simulink model "test_model"  (R2022b)
settings: Solver=VariableStepAuto  StartTime=0.0  StopTime=7  RelTol=1e-3
values from neighbouring files (symbols this model uses):
  A = 1.08    [test_script.m]
  b = 0.1    [test_script.m]
  c = 0.008    [test_script.m]
  Cd = 1.02    [test_script.m]
  g = 9.81    [test_script.m]
  gr = 47/13    (= 3.61538461538)    [test_script.m]
  h_cg = .259    (= 0.259)    [test_script.m]
  h_d = h_cg    (= 0.259)    [test_script.m]
  J = 0.27    [test_script.m]
  m = 297    [test_script.m]
  r = 0.5588    [test_script.m]
  rho = 1.162    [test_script.m]
  wb = 1.53    [test_script.m]
  wb_f = 0.813    [test_script.m]
libraries: dspswit3 x2, slpidlib x1
settings Model: Creator=sahil  LastModifiedBy=PC
settings ModelReferenceCC: EnableRefExpFcnMdlSchedulingChecks=on

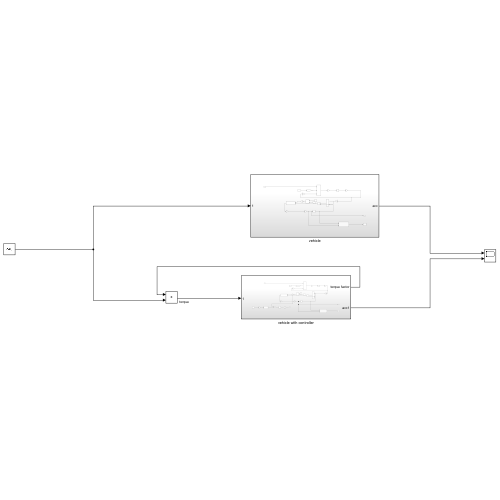
[thumbnail: Simulink's stored preview of the top-level diagram]
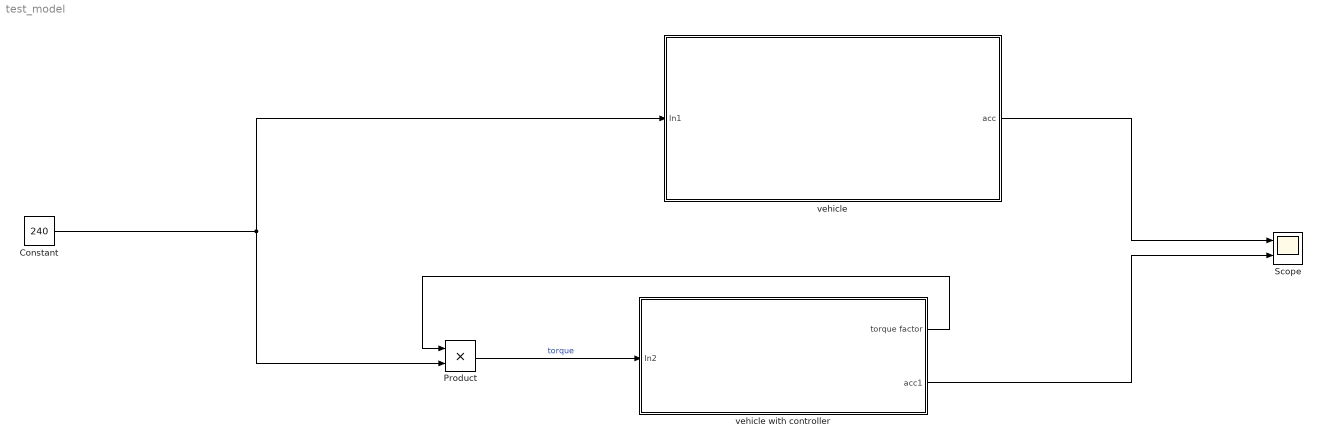
== system test_model ==
  Constant : Constant  Value=240
  Product : Product
  Scope : Scope  NumInputPorts=2
  vehicle : Subsystem
  vehicle with controller : Subsystem
  wires:
  Constant/1 -> vehicle/1(In1), Product/2
  vehicle/1(acc) -> Scope/1
  vehicle with controller/2(acc1) -> Scope/2
  Product/1 -> vehicle with controller/1(In2)  "torque"
  vehicle with controller/1(torque factor) -> Product/1

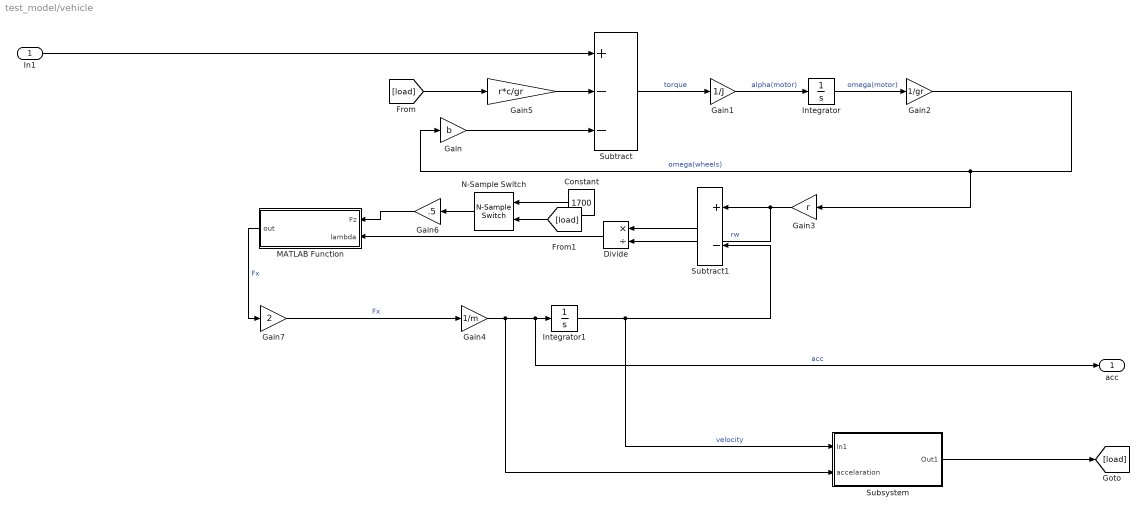
== system test_model/vehicle ==
  In1 : Inport
  Constant : Constant  Value=1700
  Divide : Product  Inputs=*/
  Gain : Gain  Gain=b
  Gain1 : Gain  Gain=1/J
  Gain2 : Gain  Gain=1/gr
  Gain3 : Gain  Gain=r
  Gain4 : Gain  Gain=1/m
  Gain5 : Gain  Gain=r*c/gr
  Gain6 : Gain  Gain=.5
  Gain7 : Gain  Gain=2
  Integrator : Integrator  InitialCondition=86.13
  Integrator1 : Integrator  InitialCondition=1
  MATLAB Function : MATLAB Function  TreatAsAtomicUnit=on
  N-Sample Switch : dspswit3/N-Sample Switch  N=1  reset=off  TriggerType=Rising edge  Ts=0.1
  Subsystem : Subsystem
  Subtract : Sum  Inputs=+--
  Subtract1 : Sum  Inputs=+-
  acc : Outport
  wires:
  Gain3/1 -> Divide/2, Subtract1/1  "rw"
  Gain/1 -> Subtract/3
  Subtract/1 -> Gain1/1  "torque"
  Gain5/1 -> Subtract/2
  Gain2/1 -> Gain3/1, Gain/1  "omega(wheels)"
  Integrator/1 -> Gain2/1  "omega(motor)"
  [load] -> Gain5/1
  Gain1/1 -> Integrator/1  "alpha(motor)"
  Integrator1/1 -> Subsystem/1(In1), Subtract1/2  "velocity"
  Divide/1 -> MATLAB Function/2(lambda)
  Subtract1/1 -> Divide/1
  Gain4/1 -> Subsystem/2(accelaration), acc/1, Integrator1/1  "acc"
  Gain7/1 -> Gain4/1  "Fx"
  Subsystem/1(Out1) -> [load]
  In1/1 -> Subtract/1
  MATLAB Function/1(out) -> Gain7/1  "Fx"
  Constant/1 -> N-Sample Switch/1
  [load] -> N-Sample Switch/2
  N-Sample Switch/1 -> Gain6/1
  Gain6/1 -> MATLAB Function/1(Fz)

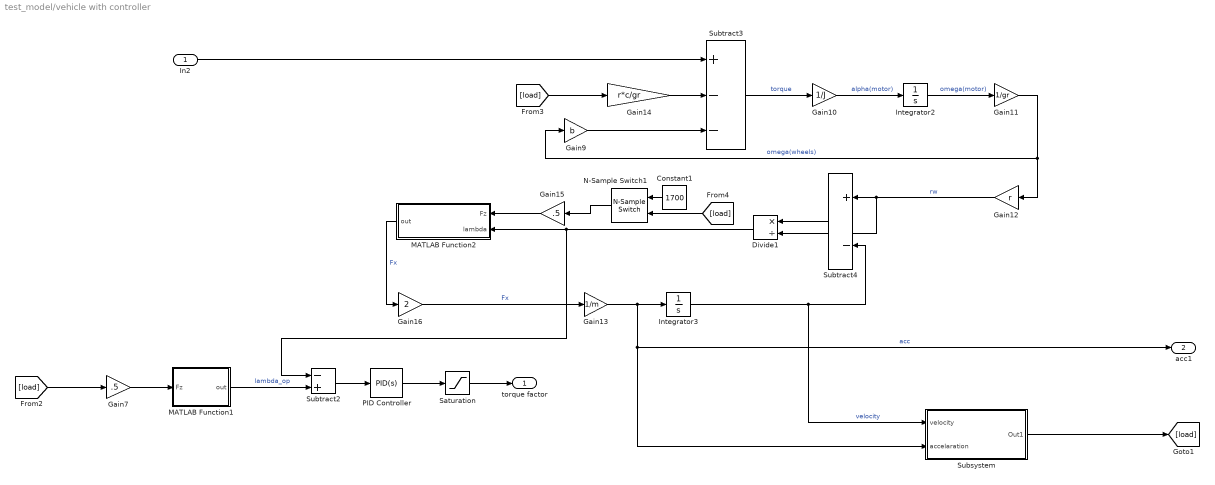
== system test_model/vehicle with controller ==
  In2 : Inport
  Constant1 : Constant  Value=1700
  Divide1 : Product  Inputs=*/
  Gain10 : Gain  Gain=1/J
  Gain11 : Gain  Gain=1/gr
  Gain12 : Gain  Gain=r
  Gain13 : Gain  Gain=1/m
  Gain14 : Gain  Gain=r*c/gr
  Gain15 : Gain  Gain=.5
  Gain16 : Gain  Gain=2
  Gain7 : Gain  Gain=.5
  Gain9 : Gain  Gain=b
  Integrator2 : Integrator  InitialCondition=86.13
  Integrator3 : Integrator  InitialCondition=1
  MATLAB Function1 : MATLAB Function  TreatAsAtomicUnit=on
  MATLAB Function2 : MATLAB Function  TreatAsAtomicUnit=on
  N-Sample Switch1 : dspswit3/N-Sample Switch  N=1  reset=off  TriggerType=Rising edge  Ts=0.1
  PID Controller : slpidlib/PID Controller  Controller=PID  Form=Parallel  TimeDomain=Continuous-time  UseExternalTs=off  SampleTime=-1  IntegratorMethod=Forward Euler  FilterMethod=Forward Euler  ControllerParametersSource=internal  P=0  I=0  UseKiTs=off  D=162.3542  N=30  UseFilter=on  TunerSelectOption=Frequency Response Based  InitialConditionSource=internal  InitialConditionForIntegrator=0  InitialConditionForFilter=0  DifferentiatorICPrevScaledInput=0  ExternalReset=none  TrackingMode=off  Kt=1  LimitOutput=off  SatLimitsSource=internal  UpperSaturationLimit=inf  LowerSaturationLimit=-inf  LinearizeAsGain=on  AntiWindupMode=none  Kb=1  LimitIntegrator=off  UpperIntegratorSaturationLimit=inf  LowerIntegratorSaturationLimit=-inf  POutMin=[]  POutMax=[]  IOutMin=[]  IOutMax=[]  DOutMin=[]  DOutMax=[]  NOutMin=[]  NOutMax=[]  SumOutMin=[]  SumOutMax=[]  SaturationOutMin=[]  SaturationOutMax=[]  PParamMin=[]  PParamMax=[]  IParamMin=[]  IParamMax=[]  DParamMin=[]  DParamMax=[]  NParamMin=[]  NParamMax=[]  KbParamMin=[]  KbParamMax=[]  KtParamMin=[]  KtParamMax=[]  KbOutMin=[]  KbOutMax=[]  KtOutMin=[]  KtOutMax=[]  IntegratorOutMin=[]  IntegratorOutMax=[]  FilterOutMin=[]  FilterOutMax=[]  SumI1OutMin=[]  SumI1OutMax=[]  SumI2OutMin=[]  SumI2OutMax=[]  SumI3OutMin=[]  SumI3OutMax=[]  SumI4OutMin=[]  SumI4OutMax=[]  SumDOutMin=[]  SumDOutMax=[]  DifferentiatorOutMin=[]  DifferentiatorOutMax=[]  FilterDiffOutCoefMin=[]  FilterDiffOutCoefMax=[]  ReciprocalOutMin=[]  ReciprocalOutMax=[]  SumDenOutMin=[]  SumDenOutMax=[]  SumNumOutMin=[]  SumNumOutMax=[]  DivideOutMin=[]  DivideOutMax=[]  UdiffTsProdOutMin=[]  UdiffTsProdOutMax=[]  NTsProdOutMin=[]  NTsProdOutMax=[]  UintegralTsProdOutMin=[]  UintegralTsProdOutMax=[]  UngainTsProdOutMin=[]  UngainTsProdOutMax=[]  ClampingZeroOutDataTypeStr=Inherit: Inherit via back propagation  ClampingZeroOutMin=[]  ClampingZeroOutMax=[]  FilterDenConstantOutDataTypeStr=Inherit: Inherit via back propagation  FilterDenConstantOutMin=[]  FilterDenConstantOutMax=[]  PCopyOutDataTypeStr=Inherit: Inherit via back propagation  PCopyOutMin=[]  PCopyOutMax=[]  NCopyOutDataTypeStr=Inherit: Inherit via back propagation  NCopyOutMin=[]  NCopyOutMax=[]  IntegratorContinuousStateAttributes=''  IntegratorStateMustResolveToSignalObject=off  IntegratorRTWStateStorageClass=Auto  FilterContinuousStateAttributes=''  FilterStateMustResolveToSignalObject=off  FilterRTWStateStorageClass=Auto  ParallelPVariant=InternalParameters  IdealPVariant=Disabled  IVariant=InternalParameters  DVariant=InternalParameters  IntegratorVariant=Continuous  SatVariant=Disabled  AWVariant=Passthrough  PCopyVariant=Disabled  TRVariant=Disabled  FdbkBlocksVariant=Forward  IdealPFdbkVariant=Disabled  SatFdbkVariant=Disabled  DerivativeFilterVariant=ContFilter  NVariant=InternalParameters  NCopyVariant=Disabled  FilterICVariant=InternalICsFilter  IntegratorICVariant=InternalICs  ExternalResetVariant=Disabled  TRSumVariant=Passthrough  SumFdbkVariant=Disabled  SumVariant=Sum_PID  TsampFilterVariant=InternalTs  TsampNgainVariant=Passthrough  TsampIntegralVariant=Passthrough  ExternalSaturationOutDataTypeStr=Inherit: Same as second input
  Saturation : Saturate  UpperLimit=1  LowerLimit=0
  Subsystem : Subsystem
  Subtract2 : Sum  Inputs=-+
  Subtract3 : Sum  Inputs=+--
  Subtract4 : Sum  Inputs=+-
  torque factor : Outport
  acc1 : Outport  Port=2
  wires:
  [load] -> Gain7/1
  MATLAB Function1/1(out) -> Subtract2/2  "lambda_op"
  Saturation/1 -> torque factor/1
  Gain7/1 -> MATLAB Function1/1(Fz)
  N-Sample Switch1/1 -> Gain15/1
  MATLAB Function2/1(out) -> Gain16/1  "Fx"
  [load] -> Gain14/1
  Integrator3/1 -> Subsystem/1(velocity), Subtract4/2  "velocity"
  Gain13/1 -> acc1/1, Subsystem/2(accelaration), Integrator3/1  "acc"
  Subtract4/1 -> Divide1/1
  Divide1/1 -> Subtract2/1, MATLAB Function2/2(lambda)
  Integrator2/1 -> Gain11/1  "omega(motor)"
  Subsystem/1(Out1) -> [load]
  Subtract3/1 -> Gain10/1  "torque"
  In2/1 -> Subtract3/1
  Gain9/1 -> Subtract3/3
  Gain10/1 -> Integrator2/1  "alpha(motor)"
  Gain16/1 -> Gain13/1  "Fx"
  Gain11/1 -> Gain12/1, Gain9/1  "omega(wheels)"
  Gain14/1 -> Subtract3/2
  Gain12/1 -> Divide1/2, Subtract4/1  "rw"
  Gain15/1 -> MATLAB Function2/1(Fz)
  Constant1/1 -> N-Sample Switch1/1
  [load] -> N-Sample Switch1/2
  PID Controller/1 -> Saturation/1
  Subtract2/1 -> PID Controller/1

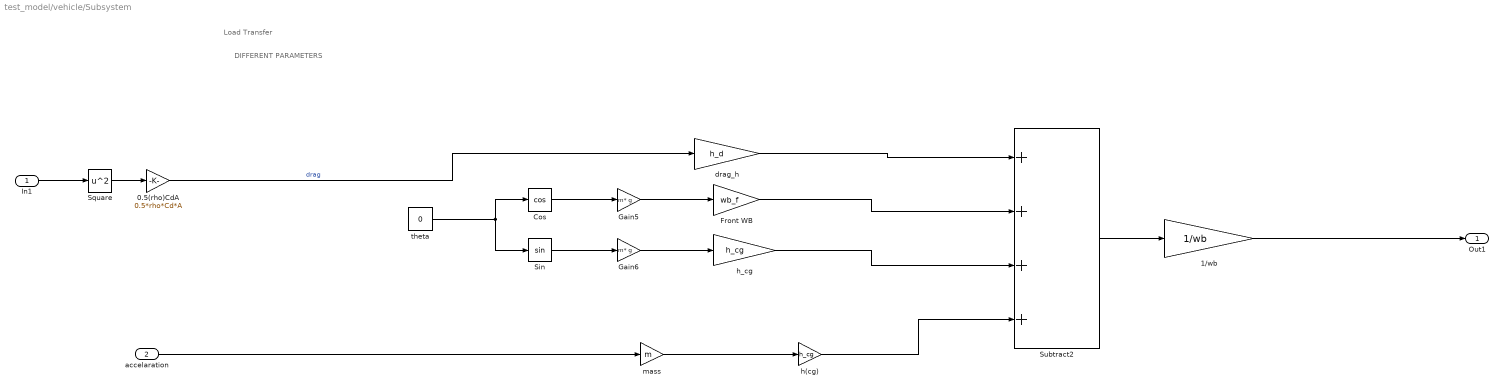
== system test_model/vehicle/Subsystem ==
  note: Load Transfer
  note: DIFFERENT PARAMETERS
  In1 : Inport
  accelaration : Inport  Port=2
  0.5(rho)CdA : Gain  Gain=0.5*rho*Cd*A
  1/wb : Gain  Gain=1/wb
  Cos : Trigonometry  Operator=cos
  Front WB : Gain  Gain=wb_f
  Gain5 : Gain  Gain=m* g
  Gain6 : Gain  Gain=m* g
  Sin : Trigonometry
  Square : Math  Operator=square
  Subtract2 : Sum  Inputs=++++
  drag_h : Gain  Gain=h_d
  h(cg) : Gain  Gain=h_cg
  h_cg : Gain  Gain=h_cg
  mass : Gain  Gain=m
  theta : Constant  Value=0
  Out1 : Outport
  wires:
  Cos/1 -> Gain5/1
  Gain6/1 -> h_cg/1
  theta/1 -> Sin/1, Cos/1
  0.5(rho)CdA/1 -> drag_h/1  "drag"
  Subtract2/1 -> 1/wb/1
  accelaration/1 -> mass/1
  drag_h/1 -> Subtract2/1
  h_cg/1 -> Subtract2/3
  Sin/1 -> Gain6/1
  Gain5/1 -> Front WB/1
  h(cg)/1 -> Subtract2/4
  Front WB/1 -> Subtract2/2
  Square/1 -> 0.5(rho)CdA/1
  mass/1 -> h(cg)/1
  1/wb/1 -> Out1/1
  In1/1 -> Square/1

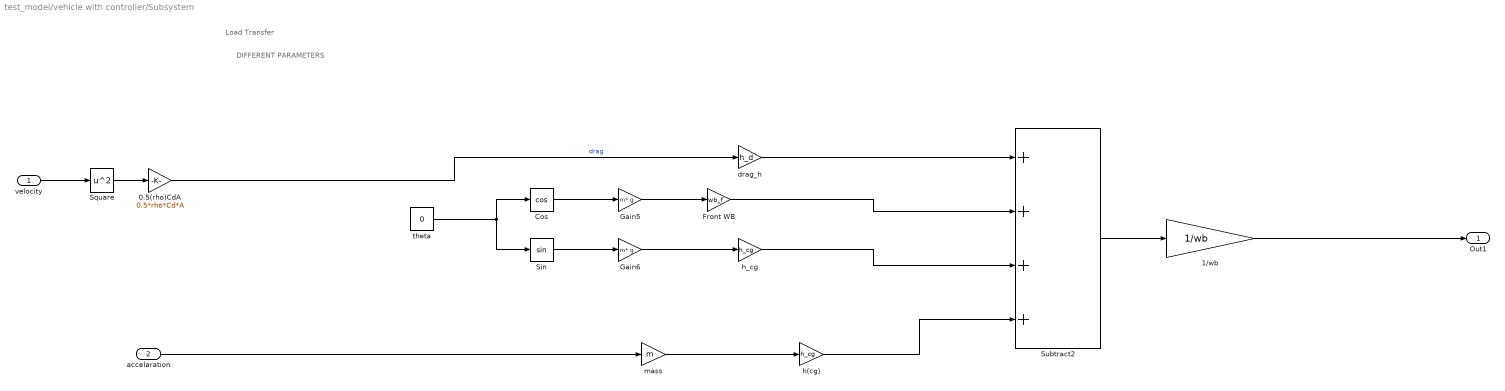
== system test_model/vehicle with controller/Subsystem ==
  note: Load Transfer
  note: DIFFERENT PARAMETERS
  velocity : Inport
  accelaration : Inport  Port=2
  0.5(rho)CdA : Gain  Gain=0.5*rho*Cd*A
  1/wb : Gain  Gain=1/wb
  Cos : Trigonometry  Operator=cos
  Front WB : Gain  Gain=wb_f
  Gain5 : Gain  Gain=m* g
  Gain6 : Gain  Gain=m* g
  Sin : Trigonometry
  Square : Math  Operator=square
  Subtract2 : Sum  Inputs=++++
  drag_h : Gain  Gain=h_d
  h(cg) : Gain  Gain=h_cg
  h_cg : Gain  Gain=h_cg
  mass : Gain  Gain=m
  theta : Constant  Value=0
  Out1 : Outport
  wires:
  Cos/1 -> Gain5/1
  Gain6/1 -> h_cg/1
  theta/1 -> Sin/1, Cos/1
  0.5(rho)CdA/1 -> drag_h/1  "drag"
  Subtract2/1 -> 1/wb/1
  accelaration/1 -> mass/1
  drag_h/1 -> Subtract2/1
  h_cg/1 -> Subtract2/3
  Sin/1 -> Gain6/1
  Gain5/1 -> Front WB/1
  h(cg)/1 -> Subtract2/4
  Front WB/1 -> Subtract2/2
  Square/1 -> 0.5(rho)CdA/1
  mass/1 -> h(cg)/1
  1/wb/1 -> Out1/1
  velocity/1 -> Square/1

== matlab function test_model/vehicle with controller/MATLAB Function1 ==
  data: Fz input; out output
function out=packeja(Fz)
    
    a1=-2.13*(10^-5);
    a2=1.144;
    a3=4.96*(10^-5);
    a4=.226;
    a5=6.9*(10^-5);
    a6=-6*(10^-9);
    a7=5.6*(10*(-5));
    a8=.486;
    
    lambda=0:.005:1;
    Cx=1.65;
    Dx=a1*Fz*Fz+a2*Fz;
    func1=(a3*Fz*Fz+a4*Fz)*exp(-a5*Fz);
    Bx=func1/(Cx*Dx);
    Ex=a6*Fz*Fz+a7*Fz+a8;
    G=Bx*lambda;
    func2=G*(1-Ex)+Ex*atan(G);
    Fx=Dx*sin(Cx*atan(func2));
    plot(lambda,Fx)
    [~,I]=max(Fx);
    slip=lambda(I);
    out=slip;

end

== matlab function test_model/vehicle with controller/MATLAB Function2 ==
  data: Fz input; out output; lambda input
function out=force(Fz,lambda)
    
    
    a1=-2.13*(10^-5);
    a2=1.144;
    a3=4.96*(10^-5);
    a4=.226;
    a5=6.9*(10^-5);
    a6=-6*(10^-9);
    a7=5.6*(10*(-5));
    a8=.486;
    
    
    Cx=1.65;
    Dx=a1*Fz*Fz+a2*Fz;
    func1=(a3*Fz*Fz+a4*Fz)*exp(-a5*Fz);
    Bx=func1/(Cx*Dx);
    Ex=a6*Fz*Fz+a7*Fz+a8;
    G=Bx*lambda;
    func2=G*(1-Ex)+Ex*atan(G);
    Fx=Dx*sin(Cx*atan(func2));
    out = Fx;
end

== matlab function test_model/vehicle/MATLAB Function ==
  data: Fz input; out output; lambda input
function out=force(Fz,lambda)
    
    
    a1=-2.13*(10^-5);
    a2=1.144;
    a3=4.96*(10^-5);
    a4=.226;
    a5=6.9*(10^-5);
    a6=-6*(10^-9);
    a7=5.6*(10*(-5));
    a8=.486;
    
    
    Cx=1.65;
    Dx=a1*Fz*Fz+a2*Fz;
    func1=(a3*Fz*Fz+a4*Fz)*exp(-a5*Fz);
    Bx=func1/(Cx*Dx);
    Ex=a6*Fz*Fz+a7*Fz+a8;
    G=Bx*lambda;
    func2=G*(1-Ex)+Ex*atan(G);
    Fx=Dx*sin(Cx*atan(func2));
    out = Fx;
end
